simulink model "chap4_9sim"  (Simulink 3.00)
settings: Solver=ode45  StartTime=0.0  StopTime=10  RelTol=1e-3
settings Model: LastModifiedBy=liu

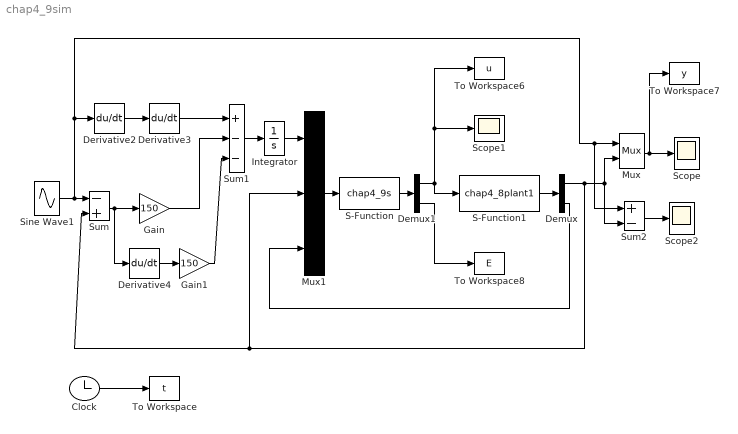
== system chap4_9sim ==
  Clock : Clock
  Demux : Demux  Outputs=2
  Demux1 : Demux  Outputs=2
  Derivative2 : Derivative
  Derivative3 : Derivative
  Derivative4 : Derivative
  Gain : Gain  Gain=150  SaturateOnIntegerOverflow=on
  Gain1 : Gain  Gain=150  SaturateOnIntegerOverflow=on
  Integrator : Integrator  ExternalReset=none  InitialConditionSource=internal  InitialCondition=0  LimitOutput=off  UpperSaturationLimit=inf  LowerSaturationLimit=-inf  ShowSaturationPort=off  ShowStatePort=off  AbsoluteTolerance=auto
  Mux : Mux  Inputs=2
      settings: DisplayOption=none
  Mux1 : Mux  Inputs=3
      settings: DisplayOption=none
  S-Function : S-Function  FunctionName=chap4_9s  PortCounts=[]  SFunctionModules=''
  S-Function1 : S-Function  FunctionName=chap4_8plant1  PortCounts=[]  SFunctionModules=''
  Scope : Scope
      settings: TimeRange=3  YMin=-0.225  YMax=0.2  SaveToWorkspace=off  SaveName=ScopeData  MaxRows=500000
  Scope1 : Scope
      settings: TimeRange=3  YMin=-0.1  YMax=0.13  SaveToWorkspace=off  SaveName=ScopeData  MaxRows=500000
  Scope2 : Scope
      settings: TimeRange=3  YMin=-1  YMax=1  SaveToWorkspace=off  SaveName=ScopeData  MaxRows=500000
  Sine Wave1 : Sin  Amplitude=0.2  Frequency=pi  Phase=pi/2  SampleTime=0
  Sum : Sum  Inputs=-+  SaturateOnIntegerOverflow=on
  Sum1 : Sum  Inputs=+--  SaturateOnIntegerOverflow=on
  Sum2 : Sum  Inputs=+-  SaturateOnIntegerOverflow=on
  To Workspace : ToWorkspace  VariableName=t  SampleTime=-1  SaveFormat=Matrix
  To Workspace6 : ToWorkspace  VariableName=u  SampleTime=-1  SaveFormat=Matrix
  To Workspace7 : ToWorkspace  VariableName=y  SampleTime=-1  SaveFormat=Matrix
  To Workspace8 : ToWorkspace  VariableName=E  SampleTime=-1  SaveFormat=Matrix
  wires:
  Derivative4/1 -> Gain1/1
  Sine Wave1/1 -> Sum/1, Derivative2/1, Mux/1, Sum2/1
  Sum/1 -> Gain/1, Derivative4/1
  Derivative2/1 -> Derivative3/1
  Derivative3/1 -> Sum1/1
  Gain/1 -> Sum1/2
  Gain1/1 -> Sum1/3
  Clock/1 -> To Workspace/1
  Mux1/1 -> S-Function/1
  Integrator/1 -> Mux1/1
  Sum1/1 -> Integrator/1
  S-Function/1 -> Demux1/1
  Mux/1 -> Scope/1, To Workspace7/1
  Demux/1 -> Mux/2, Sum2/2, Sum/2, Mux1/2
  S-Function1/1 -> Demux/1
  Demux/2 -> Mux1/3
  Demux1/1 -> S-Function1/1, Scope1/1, To Workspace6/1
  Demux1/2 -> To Workspace8/1
  Sum2/1 -> Scope2/1
